simulink model "piezo"  (R2021b)
settings: Solver=VariableStepAuto  StartTime=0.0  StopTime=1  RelTol=1e-3
values from neighbouring files (symbols this model uses):
  A1 = 1 / (1 + K)    [init_para.m]
  A11 = 1 / (1+2*K+K^2)    [init_para.m]
  A111 = (1+V)/4    (= 0.25125)    [init_para.m]
  A2 = K / (1 + K)    [init_para.m]
  A22 = 2 * K / (1+2*K+K^2)    [init_para.m]
  A222 = (1-V)/2    (= 0.4975)    [init_para.m]
  A33 = K^2 / (1+2*K+K^2)    [init_para.m]
  A333 = (1+V)/4    (= 0.25125)    [init_para.m]
  t2 = pi / w_n    [init_para.m]
  td = pi / (w_n * sqrt(1 - zeta^2))    [init_para.m]
  td1 = td    [init_para.m]
  td2 = 2 * td    [init_para.m]
  w_n = pi / (tp * sqrt(1 - zeta^2))    [init_para.m]
  zeta = log(1/Mp) / sqrt(pi^2 + (log(1/Mp))^2)    [init_para.m]
settings Model: Creator=28626  LastModifiedBy=28626

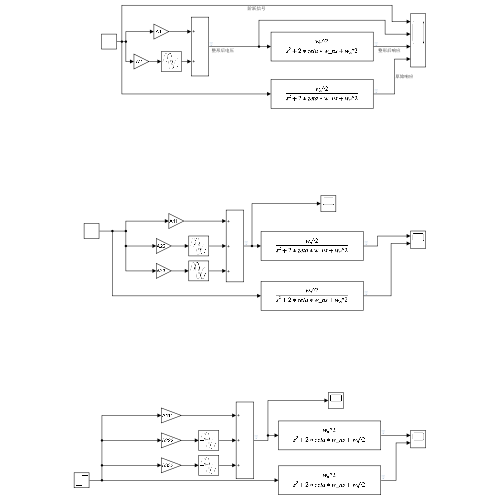
[thumbnail: Simulink's stored preview of the top-level diagram]
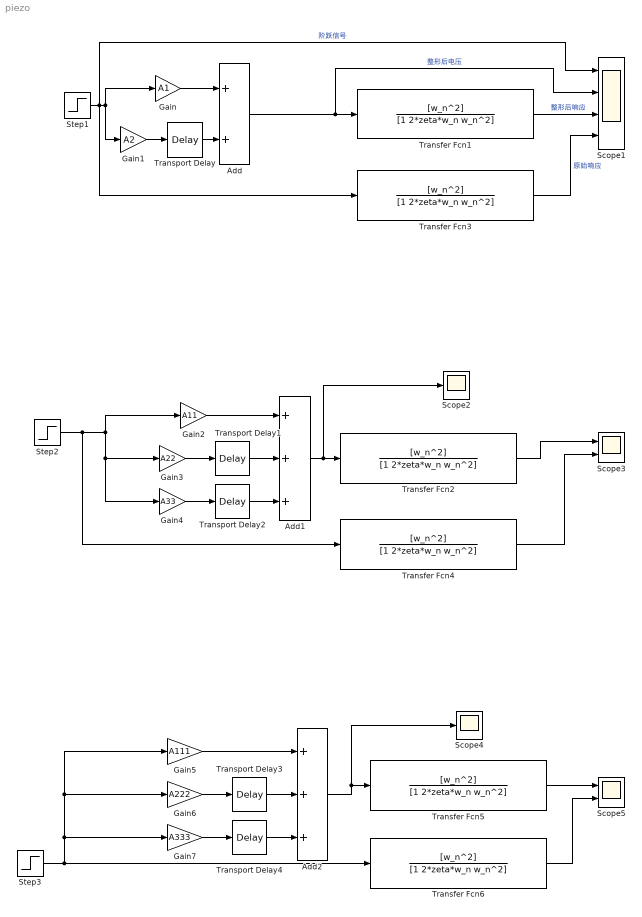
== system piezo ==
  Add : Sum
  Add1 : Sum  Inputs=+++
  Add2 : Sum  Inputs=+++
  Gain : Gain  Gain=A1
  Gain1 : Gain  Gain=A2
  Gain2 : Gain  Gain=A11
  Gain3 : Gain  Gain=A22
  Gain4 : Gain  Gain=A33
  Gain5 : Gain  Gain=A111
  Gain6 : Gain  Gain=A222
  Gain7 : Gain  Gain=A333
  Scope1 : Scope  NumInputPorts=4
  Scope2 : Scope
  Scope3 : Scope  NumInputPorts=2
  Scope4 : Scope
  Scope5 : Scope  NumInputPorts=2
  Step1 : Step  Time=0.5  After=8  SampleTime=0
  Step2 : Step  Time=0.5  After=8  SampleTime=0
  Step3 : Step  Time=0.5  After=8  SampleTime=0
  Transfer Fcn{1..6} (6 alike) : TransferFcn  Numerator=[w_n^2]  Denominator=[1 2*zeta*w_n w_n^2]
  Transport Delay : TransportDelay  DelayTime=td  PadeOrder=1
  Transport Delay1 : TransportDelay  DelayTime=td1  PadeOrder=1
  Transport Delay2 : TransportDelay  DelayTime=td2  PadeOrder=1
  Transport Delay3 : TransportDelay  DelayTime=t2  PadeOrder=1
  Transport Delay4 : TransportDelay  DelayTime=2*t2  PadeOrder=1
  wires:
  Transfer Fcn3/1 -> Scope1/4  "原始响应"
  Transfer Fcn1/1 -> Scope1/3  "整形后响应"
  Transport Delay/1 -> Add/2
  Gain/1 -> Add/1
  Gain1/1 -> Transport Delay/1
  Step1/1 -> Transfer Fcn3/1, Scope1/1, Gain1/1, Gain/1  "阶跃信号"
  Gain3/1 -> Transport Delay1/1
  Add1/1 -> Scope2/1, Transfer Fcn2/1
  Transport Delay1/1 -> Add1/2
  Transfer Fcn2/1 -> Scope3/1
  Transfer Fcn4/1 -> Scope3/2
  Gain2/1 -> Add1/1
  Transport Delay2/1 -> Add1/3
  Step2/1 -> Transfer Fcn4/1, Gain4/1, Gain3/1, Gain2/1
  Gain4/1 -> Transport Delay2/1
  Step3/1 -> Transfer Fcn6/1, Gain5/1, Gain6/1, Gain7/1
  Gain7/1 -> Transport Delay4/1
  Gain6/1 -> Transport Delay3/1
  Transfer Fcn5/1 -> Scope5/1
  Transport Delay4/1 -> Add2/3
  Transport Delay3/1 -> Add2/2
  Add2/1 -> Scope4/1, Transfer Fcn5/1
  Transfer Fcn6/1 -> Scope5/2
  Gain5/1 -> Add2/1
  Add/1 -> Scope1/2, Transfer Fcn1/1  "整形后电压"
